simulink model "DualActiveBridge_VpCntWithPIDAutoTuner"  (R2023b)
settings: Solver=ode23t  StartTime=0.0  StopTime=0.8  MaxStep=Tsw/50  RelTol=1e-3  AbsTol=1e-3
PreLoadFcn:
  | DAB_DesignSheet
undefined symbols (not defined in the file): p, Tlpf, Tsw
libraries: fl_lib x3, slpidlib x2, nesl_utility x2, slctrl_autotuning x1
settings Model: Creator=ykamatan  LastModifiedBy=ykamatan
settings SolverCC: AutoScaleAbsTol=off  AlgebraicLoopSolver=TrustRegion
settings DebuggingCC: UnconnectedInputMsg=warning  UnconnectedOutputMsg=warning  UnconnectedLineMsg=warning  SymbolicDimsDataTypeCodeGenerationDiagnostic=none
settings ModelReferenceCC: EnableRefExpFcnMdlSchedulingChecks=on
settings SFSimCC: CustomCodeUndefinedFunction=UseInterfaceOnly
settings RTWCC: DLArmComputeVersion=19.05
settings SimscapeCC: SimscapeLogType=local  SimscapeLogSimulationStatistics=on  SimscapeLogToSDI=on  SimscapeLogLimitData=off  SimscapeLogDataHistory=10000

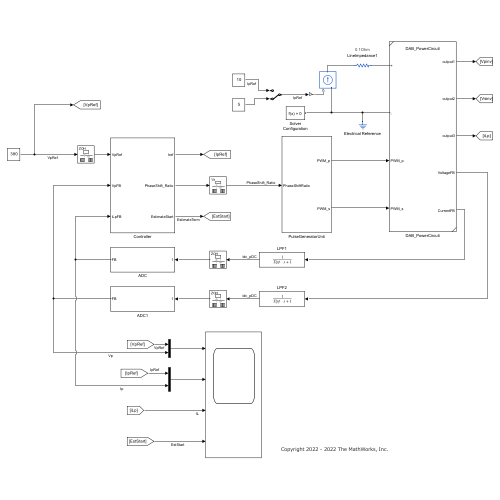
[thumbnail: Simulink's stored preview of the top-level diagram]
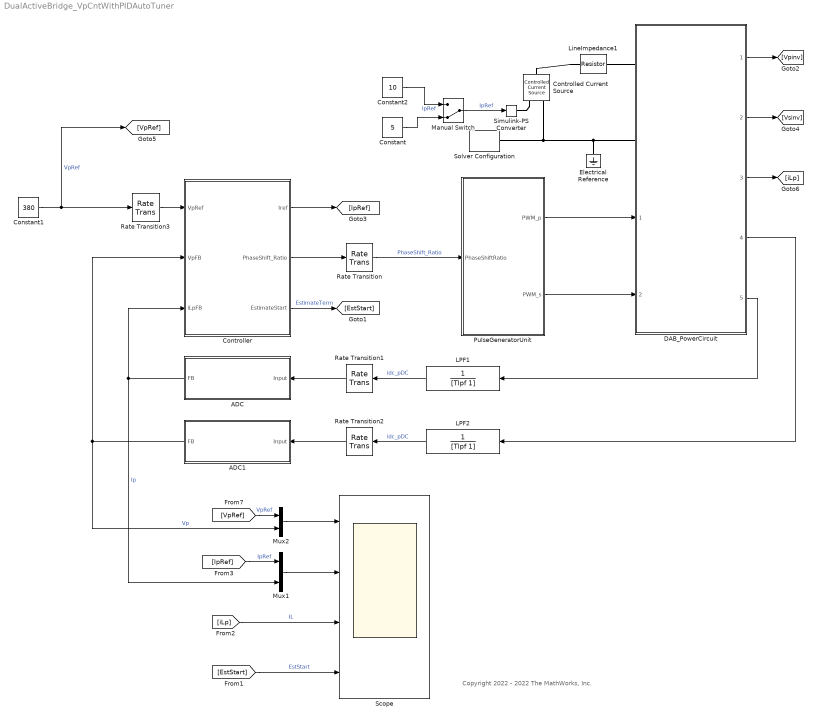
== system DualActiveBridge_VpCntWithPIDAutoTuner ==
  note: Copyright 2022 - 2022 The MathWorks, Inc.
  ADC : Subsystem
  ADC1 : Subsystem
  Constant : Constant  Value=5
  Constant1 : Constant  Value=380
  Constant2 : Constant  Value=10
  Controlled Current Source : fl_lib/Electrical/Electrical Sources/Controlled Current Source
  Controller : Subsystem
  DAB_PowerCircuit : Subsystem  ReferencedSubsystem=DAB_PowerCircuit
      settings: PortSchema="{\"entries\":[{\"content\":{\"sides\":[{\"content\":{\"connectorIds\":[\"LConn1\",\"LConn2\",\"In1\",\"In2\"]},\"type\":\"ConnectorPlacement.EquallySpacedRectSide\",\"uuid\":\"828afb30-019f-4264-8411-bc10d9e5858c\"},{\"content\":{\"connectorIds\":[\"Out1\",\"Out2\",\"Out3\",\"Out4\",\"Out5\"],\"side\":\"RIGHT\"},\"type\":\"ConnectorPlacement.EquallySpacedRectSide\",\"uuid\":\"a5597028-647d-41f2-8613-0737d9d532dd\"},{\"content\":{\"side\":\"TOP\"},\"type\":\"ConnectorPlacement.EquallySpacedRectSide\",\"uuid\":\"63db0c14-b0cf-4af7-b0f6-89f3f0342ca0\"},{\"content\":{\"side\":\"BOTTOM\"},\"type\":\"ConnectorPlacement.EquallySpacedRectSide\",\"uuid\":\"8271aac7-9cea-425f-8ea3-bca48cddb024\"}]},\"type\":\"ConnectorPlacement.EquallySpacedConnector\",\"uuid\":\"a2e479ac-6dd7-4178-b592-9d059eb37ee2\"}],\"packageUris\":[\"http://schema.mathworks.com/mf0/Connector/R2020b\"],\"version\":\"1.0\"}"
  Electrical Reference : fl_lib/Electrical/Electrical Elements/Electrical Reference
  LPF1 : TransferFcn  Denominator=[Tlpf 1]
  LPF2 : TransferFcn  Denominator=[Tlpf 1]
  LineImpedance1 : fl_lib/Electrical/Electrical Elements/Resistor  R=0.1 Ohm  i_specify=off  i_priority=None  i=0 A  i_nominal_specify=off  i_nominal_unit=A  i_nominal_value=1  v_specify=off  v_priority=None  v=0 V  v_nominal_specify=off  v_nominal_unit=V  v_nominal_value=1
      settings: AttributesFormatString=%<R>%<R_unit>  LogSimulationData=on
  Manual Switch : ManualSwitch  CurrentSetting=0
  Mux1 : Mux  Inputs=2
  Mux2 : Mux  Inputs=2
  PulseGeneratorUnit : Subsystem
  Rate Transition{,1..3} (4 alike) : RateTransition
  Scope : Scope  NumInputPorts=4
  Simulink-PS Converter : nesl_utility/Simulink-PS Converter  PhysicalDomain=network_engine_domain  SubClassName=ps_input  LeftPortType=input  RightPortType=output  PseudoPeriodic=off  Frequencies=[]  NoiseDistribution=none  NoiseParameters=[]  Unit=1  AffineConversion=off  FilteringAndDerivatives=provide  SimscapeFilterOrder=1  InputFilterTimeConstant=0.001  UdotUserProvided=0
  Solver Configuration : nesl_utility/Solver Configuration  PhysicalDomain=network_engine_domain  SubClassName=solver  LeftPortType=input  RightPortType=generic  Tones=[]  Harmonics=[]  SimulateNoise=off  Profile=off  UseLocalSampling=off  EnableSwitchedLinearOptims=on  FrequencyDomain=off  UseCCode=off  RelTol=0.001  AbsTol=1e-06  MinStep=1e-09  ToWorkspace=off  RevertToSquareIcSolve=off  NumHomotopyIterations=100  PhasorMode=off  PhasorModeNumHarmonics=1  ConsistencySolver=NEWTON_XTOL_AFTER_FTOL  IndexReductionMethod=DerivativeReplacement  DoDC=off  ResidualTolerance=1e-09  ConsistencyTolSource=GLOBAL  ConsistencyAbsTol=0.001  ConsistencyRelTol=0.001  ConsistencyTolFactor=0.001  UseLocalSolver=off  LocalSolverChoice=NE_BACKWARD_EULER_ADVANCER  ResolveIndetEquations=on  FunctionEvalNumThread=1  LocalSolverSampleTime=0.001  DoFixedCost=off  MaxNonlinIter=3  MaxModeIter=2  ComputeImpulses=off  ImpulseIterations=2  LinearAlgebra=auto  LinearAlgebraNumThread=0  EquationFormulation=NE_TIME_EF  DelaysMemoryBudget=1024  AutomaticFiltering=on  FilteringTimeConstant=0.001  PartitionStorageMethod=AS_NEEDED  PartitionMemoryBudget=1024  PartitionMethod=ROBUST  MultibodyUseLocalSolver=off  MultibodyLocalSolverChoice=ODE1  MultibodyLocalSolverSampleTime=0.001
  wires:
  Rate Transition/1 -> PulseGeneratorUnit/1(PhaseShiftRatio)  "PhaseShift_Ratio"
  Mux1/1 -> Scope/2
  [iLp] -> Scope/3  "IL"
  Manual Switch/1 -> Simulink-PS Converter/1  "IpRef"
  [IpRef] -> Mux1/1  "IpRef"
  ADC1/1(FB) -> Controller/2(VpFB), Mux2/2  "Vp"
  Constant1/1 -> [VpRef], Rate Transition3/1  "VpRef"
  ADC/1(FB) -> Mux1/2, Controller/3(iLpFB)  "Ip"
  Controller/1(Iref) -> [IpRef]
  Controller/2(PhaseShift_Ratio) -> Rate Transition/1
  Rate Transition3/1 -> Controller/1(VpRef)
  Mux2/1 -> Scope/1
  [VpRef] -> Mux2/1  "VpRef"
  Constant2/1 -> Manual Switch/1  "IpRef"
  Constant/1 -> Manual Switch/2
  PulseGeneratorUnit/2(PWM_s) -> DAB_PowerCircuit/2
  PulseGeneratorUnit/1(PWM_p) -> DAB_PowerCircuit/1
  Rate Transition1/1 -> ADC/1(Input)
  LPF1/1 -> Rate Transition1/1  "idc_pDC"
  Rate Transition2/1 -> ADC1/1(Input)
  LPF2/1 -> Rate Transition2/1  "idc_pDC"
  DAB_PowerCircuit/4 -> LPF2/1
  DAB_PowerCircuit/5 -> LPF1/1
  Controller/3(EstimateStart) -> [EstStart]  "EstimateTerm"
  [EstStart] -> Scope/4  "EstStart"
  DAB_PowerCircuit/1 -> [Vpinv]
  DAB_PowerCircuit/2 -> [Vsinv]
  DAB_PowerCircuit/3 -> [iLp]
  connections:
  Solver Configuration/RConn1 -- Controlled Current Source/RConn2 -- DAB_PowerCircuit/LConn2 -- Electrical Reference/LConn1
  LineImpedance1/RConn1 -- DAB_PowerCircuit/LConn1
  Simulink-PS Converter/RConn1 -- Controlled Current Source/RConn1
  LineImpedance1/LConn1 -- Controlled Current Source/LConn1

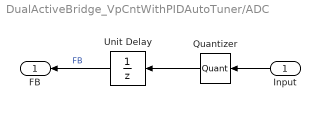
== system DualActiveBridge_VpCntWithPIDAutoTuner/ADC ==
  Input : Inport
  Quantizer : Quantizer  QuantizationInterval=0.01
  Unit Delay : UnitDelay  SampleTime=Tsw  HasFrameUpgradeWarning=on
  FB : Outport
  wires:
  Quantizer/1 -> Unit Delay/1
  Unit Delay/1 -> FB/1  "FB"
  Input/1 -> Quantizer/1

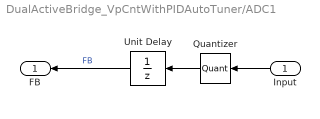
== system DualActiveBridge_VpCntWithPIDAutoTuner/ADC1 ==
  Input : Inport
  Quantizer : Quantizer  QuantizationInterval=0.01
  Unit Delay : UnitDelay  SampleTime=Tsw  HasFrameUpgradeWarning=on
  FB : Outport
  wires:
  Quantizer/1 -> Unit Delay/1
  Unit Delay/1 -> FB/1  "FB"
  Input/1 -> Quantizer/1

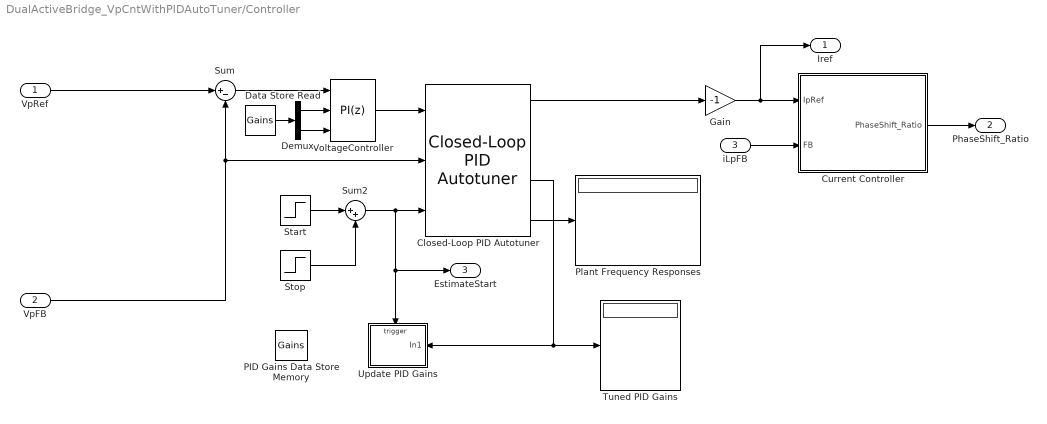
== system DualActiveBridge_VpCntWithPIDAutoTuner/Controller ==
  VpRef : Inport
  VpFB : Inport  Port=2
  iLpFB : Inport  Port=3
  Closed-Loop PID Autotuner : slctrl_autotuning/Closed-Loop PID Autotuner  PIDType=PI  PIDForm=Parallel  TimeDomain=discrete-time  DiscreteTs=Tsw  TuningTs=0.2  UseTuningTs=off  IntegratorFormula=Forward Euler  FilterFormula=Forward Euler  ContinuousTs=0.02  Bandwidth=2*pi*1000  UseExternalWC=off  TargetPM=60  UseExternalPM=off  UseExternalAchievedPM=off  ExperimentMode=Superposition  PlantType=Stable  PlantSign=Positive  AmpSine=0.3  UseExternalAmpSine=off  UseExternalFRD=on  UseExternalU0=off  UseCompanion=off  NotDeployTuningModule=off  UsePLCCoder=off  OutputMode=control action + perturbation  BlockDataType=double  UseConnectedPID=on  blockpath=[]  tunedP=0  tunedI=0  tunedD=0  tunedN=100  tunedPM=0  EstimationWindowSize=3  UseExternalTuningParams=off  SingleMultiRateVariant=SingleSamplingRate  NumEstimationPeriods=4  NumSettlingPeriods=2  NumOfPRBSPeriod=1  PRBSSignalOrder=12  ExperimentModeVariant=VariantSuperimposed  OutputChoice=VariantCandD
  Current Controller : Subsystem
  Data Store Read : DataStoreRead  DataStoreName=Gains  IndexOptions=Index vector (dialog)  Indices=1  OutputSizes=1
  Demux : Demux  Outputs=2
  Gain : Gain  Gain=-1
  PID Gains Data Store Memory : DataStoreMemory  DataStoreName=Gains  InitialValue=[2 200]  ShowAdditionalParam=off
  Plant Frequency Responses : Display
  Start : Step  Time=0.2  SampleTime=0
  Stop : Step  Time=0.5  After=-1  SampleTime=0
  Sum : Sum  Inputs=|+-
  Sum2 : Sum  Inputs=|++
  Tuned PID Gains : Display
  Update PID Gains : Subsystem
  VoltageController : slpidlib/PID Controller  Controller=PI  Form=Parallel  TimeDomain=Discrete-time  UseExternalTs=off  SampleTime=Tsw  IntegratorMethod=Forward Euler  FilterMethod=Forward Euler  ControllerParametersSource=external  P=2  I=200  UseKiTs=off  D=0  N=100  UseFilter=on  TunerSelectOption=Transfer Function Based (PID Tuner App)  InitialConditionSource=internal  InitialConditionForIntegrator=0  InitialConditionForFilter=0  DifferentiatorICPrevScaledInput=0  ExternalReset=none  TrackingMode=off  Kt=1  LimitOutput=off  SatLimitsSource=internal  UpperSaturationLimit=inf  LowerSaturationLimit=-inf  LinearizeAsGain=on  AntiWindupMode=none  Kb=1  LimitIntegrator=off  UpperIntegratorSaturationLimit=inf  LowerIntegratorSaturationLimit=-inf  POutMin=[]  POutMax=[]  IOutMin=[]  IOutMax=[]  DOutMin=[]  DOutMax=[]  NOutMin=[]  NOutMax=[]  SumOutMin=[]  SumOutMax=[]  SaturationOutMin=[]  SaturationOutMax=[]  PParamMin=[]  PParamMax=[]  IParamMin=[]  IParamMax=[]  DParamMin=[]  DParamMax=[]  NParamMin=[]  NParamMax=[]  KbParamMin=[]  KbParamMax=[]  KtParamMin=[]  KtParamMax=[]  KbOutMin=[]  KbOutMax=[]  KtOutMin=[]  KtOutMax=[]  IntegratorOutMin=[]  IntegratorOutMax=[]  FilterOutMin=[]  FilterOutMax=[]  SumI1OutMin=[]  SumI1OutMax=[]  SumI2OutMin=[]  SumI2OutMax=[]  SumI3OutMin=[]  SumI3OutMax=[]  SumI4OutMin=[]  SumI4OutMax=[]  SumDOutMin=[]  SumDOutMax=[]  DifferentiatorOutMin=[]  DifferentiatorOutMax=[]  FilterDiffOutCoefMin=[]  FilterDiffOutCoefMax=[]  ReciprocalOutMin=[]  ReciprocalOutMax=[]  SumDenOutMin=[]  SumDenOutMax=[]  SumNumOutMin=[]  SumNumOutMax=[]  DivideOutMin=[]  DivideOutMax=[]  UdiffTsProdOutMin=[]  UdiffTsProdOutMax=[]  NTsProdOutMin=[]  NTsProdOutMax=[]  UintegralTsProdOutMin=[]  UintegralTsProdOutMax=[]  UngainTsProdOutMin=[]  UngainTsProdOutMax=[]  ClampingZeroOutDataTypeStr=Inherit: Inherit via back propagation  ClampingZeroOutMin=[]  ClampingZeroOutMax=[]  FilterDenConstantOutDataTypeStr=Inherit: Inherit via back propagation  FilterDenConstantOutMin=[]  FilterDenConstantOutMax=[]  PCopyOutDataTypeStr=Inherit: Inherit via back propagation  PCopyOutMin=[]  PCopyOutMax=[]  NCopyOutDataTypeStr=Inherit: Inherit via back propagation  NCopyOutMin=[]  NCopyOutMax=[]  IntegratorContinuousStateAttributes=''  IntegratorStateMustResolveToSignalObject=off  IntegratorRTWStateStorageClass=Auto  FilterContinuousStateAttributes=''  FilterStateMustResolveToSignalObject=off  FilterRTWStateStorageClass=Auto  ParallelPVariant=ExternalParameters  IdealPVariant=Disabled  IVariant=ExternalParameters  DVariant=Disabled  IntegratorVariant=Discrete  SatVariant=Disabled  AWVariant=Passthrough  PCopyVariant=Disabled  TRVariant=Disabled  FdbkBlocksVariant=Forward  IdealPFdbkVariant=Disabled  SatFdbkVariant=Disabled  DerivativeFilterVariant=Disabled  NVariant=Disabled  NCopyVariant=Disabled_SignalSpec  FilterICVariant=Disabled  IntegratorICVariant=InternalICs  ExternalResetVariant=Disabled  TRSumVariant=Passthrough  SumFdbkVariant=Disabled  SumVariant=Sum_PI  TsampFilterVariant=InternalTs  TsampNgainVariant=Passthrough  TsampIntegralVariant=Disabled_SignalSpec  ExternalSaturationOutDataTypeStr=Inherit: Same as second input
  Iref : Outport
  PhaseShift_Ratio : Outport  Port=2
  EstimateStart : Outport  Port=3
  wires:
  VpFB/1 -> Sum/2, Closed-Loop PID Autotuner/2
  VoltageController/1 -> Closed-Loop PID Autotuner/1
  Sum/1 -> VoltageController/1
  Current Controller/1(PhaseShift_Ratio) -> PhaseShift_Ratio/1
  VpRef/1 -> Sum/1
  iLpFB/1 -> Current Controller/2(FB)
  Gain/1 -> Current Controller/1(IpRef), Iref/1
  Closed-Loop PID Autotuner/1 -> Gain/1
  Closed-Loop PID Autotuner/3 -> Update PID Gains/1(In1), Tuned PID Gains/1
  Closed-Loop PID Autotuner/4 -> Plant Frequency Responses/1
  Start/1 -> Sum2/1
  Stop/1 -> Sum2/2
  Data Store Read/1 -> Demux/1
  Demux/1 -> VoltageController/2
  Demux/2 -> VoltageController/3
  Sum2/1 -> EstimateStart/1, Update PID Gains/Trigger, Closed-Loop PID Autotuner/3

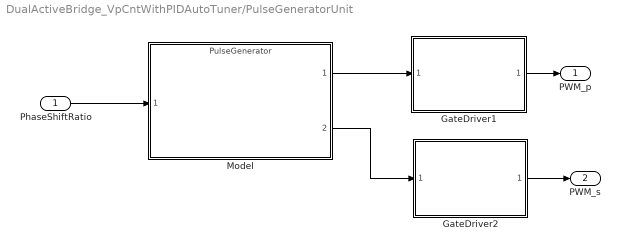
== system DualActiveBridge_VpCntWithPIDAutoTuner/PulseGeneratorUnit ==
  PhaseShiftRatio : Inport
  GateDriver1 : Subsystem  ReferencedSubsystem=GateDriver
      settings: PortSchema="{\"entries\":[{\"content\":{\"sides\":[{\"content\":{\"connectorIds\":[\"Out1\"]},\"type\":\"ConnectorPlacement.EquallySpacedRectSide\",\"uuid\":\"311475b7-00eb-40fb-907f-61918164ee7b\"},{\"content\":{\"connectorIds\":[\"In1\"],\"side\":\"RIGHT\"},\"type\":\"ConnectorPlacement.EquallySpacedRectSide\",\"uuid\":\"0b8731f7-8da9-403f-8880-992b54f942ab\"},{\"content\":{\"side\":\"TOP\"},\"type\":\"ConnectorPlacement.EquallySpacedRectSide\",\"uuid\":\"6fd0a64f-df87-43d4-a7cc-9e3ddd37bd1a\"}]},\"type\":\"ConnectorPlacement.EquallySpacedConnector\",\"uuid\":\"c1f4b631-9d66-4028-87ab-7567590c1b71\"}],\"packageUris\":[\"http://schema.mathworks.com/mf0/Connector/R2020b\"],\"version\":\"1.0\"}"
  GateDriver2 : Subsystem  ReferencedSubsystem=GateDriver
  Model : ModelReference  ModelNameDialog=PulseGenerator.slx  SimulationMode=Normal  ModelReferenceVersion=8.0
  PWM_p : Outport
  PWM_s : Outport  Port=2
  wires:
  GateDriver2/1 -> PWM_s/1
  PhaseShiftRatio/1 -> Model/1
  Model/2 -> GateDriver2/1
  Model/1 -> GateDriver1/1
  GateDriver1/1 -> PWM_p/1

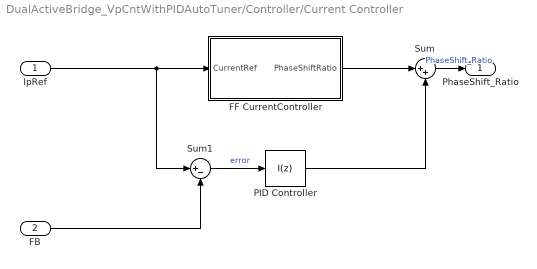
== system DualActiveBridge_VpCntWithPIDAutoTuner/Controller/Current Controller ==
  IpRef : Inport
  FB : Inport  Port=2
  FF CurrentController : Subsystem
  PID Controller : slpidlib/PID Controller  Controller=I  Form=Parallel  TimeDomain=Discrete-time  UseExternalTs=off  SampleTime=Tsw  IntegratorMethod=Forward Euler  FilterMethod=Forward Euler  ControllerParametersSource=internal  P=0.1  I=10  UseKiTs=off  D=0  N=100  UseFilter=on  TunerSelectOption=Transfer Function Based (PID Tuner App)  InitialConditionSource=internal  InitialConditionForIntegrator=0  InitialConditionForFilter=0  DifferentiatorICPrevScaledInput=0  ExternalReset=none  TrackingMode=off  Kt=1  LimitOutput=off  SatLimitsSource=internal  UpperSaturationLimit=inf  LowerSaturationLimit=-inf  LinearizeAsGain=on  AntiWindupMode=none  Kb=1  LimitIntegrator=off  UpperIntegratorSaturationLimit=inf  LowerIntegratorSaturationLimit=-inf  POutMin=[]  POutMax=[]  IOutMin=[]  IOutMax=[]  DOutMin=[]  DOutMax=[]  NOutMin=[]  NOutMax=[]  SumOutMin=[]  SumOutMax=[]  SaturationOutMin=[]  SaturationOutMax=[]  PParamMin=[]  PParamMax=[]  IParamMin=[]  IParamMax=[]  DParamMin=[]  DParamMax=[]  NParamMin=[]  NParamMax=[]  KbParamMin=[]  KbParamMax=[]  KtParamMin=[]  KtParamMax=[]  KbOutMin=[]  KbOutMax=[]  KtOutMin=[]  KtOutMax=[]  IntegratorOutMin=[]  IntegratorOutMax=[]  FilterOutMin=[]  FilterOutMax=[]  SumI1OutMin=[]  SumI1OutMax=[]  SumI2OutMin=[]  SumI2OutMax=[]  SumI3OutMin=[]  SumI3OutMax=[]  SumI4OutMin=[]  SumI4OutMax=[]  SumDOutMin=[]  SumDOutMax=[]  DifferentiatorOutMin=[]  DifferentiatorOutMax=[]  FilterDiffOutCoefMin=[]  FilterDiffOutCoefMax=[]  ReciprocalOutMin=[]  ReciprocalOutMax=[]  SumDenOutMin=[]  SumDenOutMax=[]  SumNumOutMin=[]  SumNumOutMax=[]  DivideOutMin=[]  DivideOutMax=[]  UdiffTsProdOutMin=[]  UdiffTsProdOutMax=[]  NTsProdOutMin=[]  NTsProdOutMax=[]  UintegralTsProdOutMin=[]  UintegralTsProdOutMax=[]  UngainTsProdOutMin=[]  UngainTsProdOutMax=[]  ClampingZeroOutDataTypeStr=Inherit: Inherit via back propagation  ClampingZeroOutMin=[]  ClampingZeroOutMax=[]  FilterDenConstantOutDataTypeStr=Inherit: Inherit via back propagation  FilterDenConstantOutMin=[]  FilterDenConstantOutMax=[]  PCopyOutDataTypeStr=Inherit: Inherit via back propagation  PCopyOutMin=[]  PCopyOutMax=[]  NCopyOutDataTypeStr=Inherit: Inherit via back propagation  NCopyOutMin=[]  NCopyOutMax=[]  IntegratorContinuousStateAttributes=''  IntegratorStateMustResolveToSignalObject=off  IntegratorRTWStateStorageClass=Auto  FilterContinuousStateAttributes=''  FilterStateMustResolveToSignalObject=off  FilterRTWStateStorageClass=Auto  ParallelPVariant=Disabled  IdealPVariant=Disabled  IVariant=InternalParameters  DVariant=Disabled  IntegratorVariant=Discrete  SatVariant=Disabled  AWVariant=Passthrough  PCopyVariant=Disabled  TRVariant=Disabled  FdbkBlocksVariant=Forward  IdealPFdbkVariant=Disabled  SatFdbkVariant=Disabled  DerivativeFilterVariant=Disabled  NVariant=Disabled  NCopyVariant=Disabled_SignalSpec  FilterICVariant=Disabled  IntegratorICVariant=InternalICs  ExternalResetVariant=Disabled  TRSumVariant=Passthrough  SumFdbkVariant=Disabled  SumVariant=Passthrough_I  TsampFilterVariant=InternalTs  TsampNgainVariant=Passthrough  TsampIntegralVariant=Disabled_SignalSpec  ExternalSaturationOutDataTypeStr=Inherit: Same as second input
  Sum : Sum  Inputs=|++
  Sum1 : Sum  Inputs=|+-
  PhaseShift_Ratio : Outport
  wires:
  FF CurrentController/1(PhaseShiftRatio) -> Sum/1
  IpRef/1 -> FF CurrentController/1(CurrentRef), Sum1/1
  Sum1/1 -> PID Controller/1  "error"
  FB/1 -> Sum1/2
  PID Controller/1 -> Sum/2
  Sum/1 -> PhaseShift_Ratio/1  "PhaseShift_Ratio"

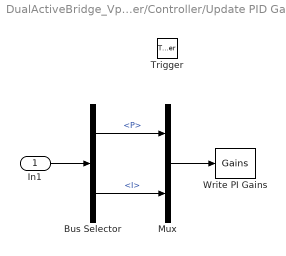
== system DualActiveBridge_VpCntWithPIDAutoTuner/Controller/Update PID Gains ==
  In1 : Inport
  Trigger : TriggerPort  TriggerType=falling  VariantControl=Variant  PortDimensions=1
  Bus Selector : BusSelector  OutputSignals=P,I
  Mux : Mux  Inputs=2
  Write PI Gains : DataStoreWrite  DataStoreName=Gains  IndexOptions=Index vector (dialog)  Indices=1  OutputSizes=1
  wires:
  In1/1 -> Bus Selector/1
  Bus Selector/1 -> Mux/1  "<P>"
  Bus Selector/2 -> Mux/2  "<I>"
  Mux/1 -> Write PI Gains/1

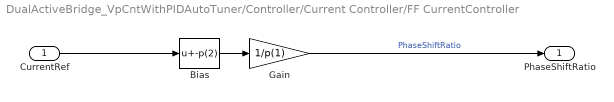
== system DualActiveBridge_VpCntWithPIDAutoTuner/Controller/Current Controller/FF CurrentController ==
  CurrentRef : Inport
  Bias : Bias  Bias=-p(2)  SaturateOnIntegerOverflow=off
  Gain : Gain  Gain=1/p(1)
  PhaseShiftRatio : Outport
  wires:
  Bias/1 -> Gain/1
  Gain/1 -> PhaseShiftRatio/1  "PhaseShiftRatio"
  CurrentRef/1 -> Bias/1
